simulink model "RmsConverterController_R2014b"  (R2014b)
settings: Solver=ode2  SolverMode=SingleTasking  StartTime=0.0  StopTime=10.0  FixedStep=2e-5  RelTol=1e-3
libraries: simulink x4, powerlib_meascontrol x2
settings Model: CovMetricSettings=dwe  CovHtmlReporting=off  covSaveCumulativeToWorkspaceVar=off  CovSaveSingleToWorkspaceVar=off  CovExternalEMLEnable=on  CovSFcnEnable=on  Creator=sandroni  LastModifiedBy=carlo
settings DataIOCC: LimitDataPoints=off  SaveFormat=StructureWithTime
settings DebuggingCC: SolverPrmCheckMsg=none  FrameProcessingCompatibilityMsg=error  SFUnexpectedBacktrackingDiag=error  SFNoUnconditionalDefaultTransitionDiag=error
settings HardwareCC: ProdBitPerPointer=64  ProdLargestAtomicFloat=Float  ProdIntDivRoundTo=Zero  ProdEndianess=LittleEndian  ProdHWDeviceType=Specified  TargetLongLongMode=on  TargetIntDivRoundTo=Zero  TargetEndianess=LittleEndian  TargetHWDeviceType=MATLAB Host  ProdEqTarget=off
settings ModelReferenceCC: PropagateSignalLabelsOutOfModel=on
settings RTWCC: SystemTargetFile=rtwsfcnfmi.tlc  TemplateMakefile=rtwsfcnfmi_tmf  Description=S-Function Target with Functional Mockup Interface (FMI)  ProcessScript=rtwsfcnfmi_make_rtw_hook
settings STFCustomTargetCC: ModelReferenceCompliant=off  CompOptLevelCompliant=on  GeneratePreprocessorConditionals=Disable all  MATLABClassNameForMDSCustomization=Simulink.SoftwareTarget.TargetSpecificTriggerConfigurationBase  SystemTargetFile=rtwsfcnfmi.tlc

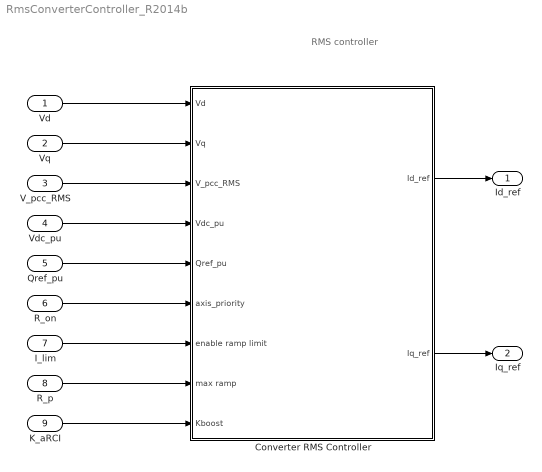
== system RmsConverterController_R2014b ==
  note: RMS controller
  Vd : Inport
  Vq : Inport  Port=2
  V_pcc_RMS : Inport  Port=3
  Vdc_pu : Inport  Port=4
  Qref_pu : Inport  Port=5
  R_on : Inport  Port=6
  I_lim : Inport  Port=7
  R_p : Inport  Port=8
  K_aRCI : Inport  Port=9
  Converter RMS Controller : Subsystem  mask(Converter RMS Controller){Kp_dc=1.1, Ki_dc=27.5, Kp_Var=1, Ki_Var=100, P0_pu=0.85, Fnom=50, Ts=2e-5}
      mask prompts: Kp_dc "DC voltage regulator proportional parameter [Kp]"; Ki_dc "DC voltage regulator integral parameter [Ki]"; Kp_Var "PCC voltage regulator proportional parameter [Kp]"; Ki_Var "PCC voltage regulator integral parameter [Ki]"; P0_pu "Initial Active Power [pu]"; Fnom "Nominal frequency [Hz]"; Ts "Sample Time [s]"
      mask init:
      | Imax_grid_conv = 1.1;
  Id_ref : Outport
  Iq_ref : Outport  Port=2
  wires:
  Qref_pu/1 -> Converter RMS Controller/5(Qref_pu)
  V_pcc_RMS/1 -> Converter RMS Controller/3(V_pcc_RMS)
  K_aRCI/1 -> Converter RMS Controller/9(Kboost)
  R_on/1 -> Converter RMS Controller/6(axis_priority)
  R_p/1 -> Converter RMS Controller/8(max ramp)
  I_lim/1 -> Converter RMS Controller/7(enable ramp limit)
  Converter RMS Controller/1(Id_ref) -> Id_ref/1
  Converter RMS Controller/2(Iq_ref) -> Iq_ref/1
  Vq/1 -> Converter RMS Controller/2(Vq)
  Vdc_pu/1 -> Converter RMS Controller/4(Vdc_pu)
  Vd/1 -> Converter RMS Controller/1(Vd)

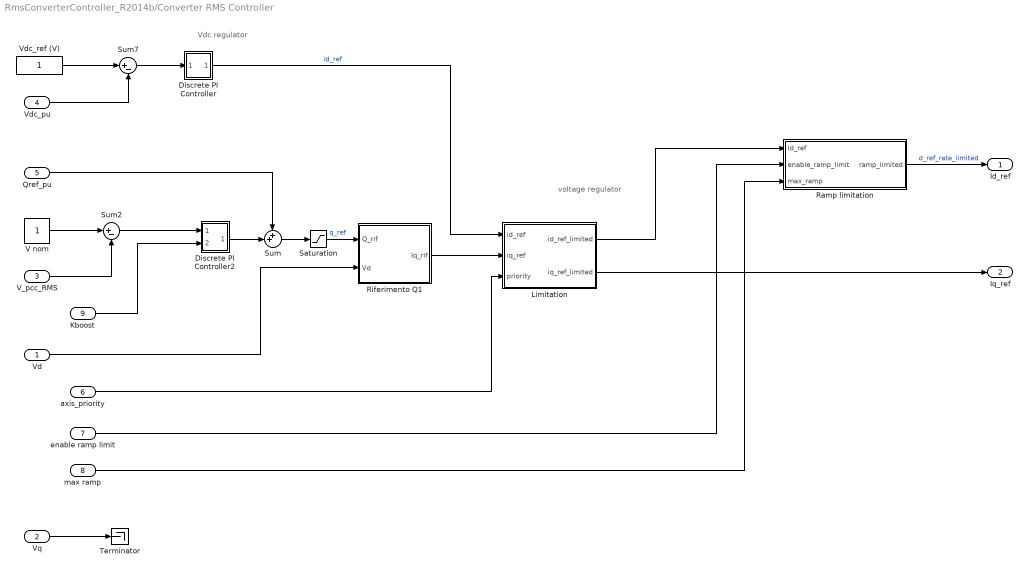
== system RmsConverterController_R2014b/Converter RMS Controller ==
  note: Vdc regulator
  note: voltage regulator
  Vd : Inport
  Vq : Inport  Port=2
  V_pcc_RMS : Inport  Port=3
  Vdc_pu : Inport  Port=4
  Qref_pu : Inport  Port=5
  axis_priority : Inport  Port=6
  enable ramp limit : Inport  Port=7
  max ramp : Inport  Port=8
  Kboost : Inport  Port=9
  Discrete PI Controller : Subsystem  DialogController=POWERSYS.PowerSysDialog  mask(Discrete PI Controller){Kp=Kp_dc, Ki=Ki_dc, Par_Limits=[1 -1]*Imax_grid_conv, Init=-P0_pu, Ts=Ts}
      mask prompts: Kp "Proportional gain (Kp):"; Ki "Integral gain (Ki):"; Par_Limits "Output limits: [ Upper   Lower ]"; Init "Output initial value:"; Ts "Sample time:"
      mask help: This block implements a discrete PI controller.
      mask init:
      | UpperLimit=Par_Limits(1);
      | LowerLimit=Par_Limits(2);
      | power_initmask();
      mask Help: This block is part of a subset of blocks in the Extras library that does not have documentation associated with it, other than the block mask description.
      mask Display: disp('PI');
  Discrete PI Controller2 : Subsystem  DialogController=POWERSYS.PowerSysDialog  mask(Discrete PI Controller){Kp=Kp_Var, Ki=Ki_Var, Par_Limits=[1 -1], Init=0, Ts=Ts}
      mask prompts: Kp "Proportional gain (Kp):"; Ki "Integral gain (Ki):"; Par_Limits "Output limits: [ Upper   Lower ]"; Init "Output initial value:"; Ts "Sample time:"
      mask help: This block implements a discrete PI controller.
      mask init:
      | UpperLimit=Par_Limits(1);
      | LowerLimit=Par_Limits(2);
      | power_initmask();
      mask Help: This block is part of a subset of blocks in the Extras library that does not have documentation associated with it, other than the block mask description.
      mask Display: disp('PI');
  Limitation : Subsystem
  Ramp limitation : Subsystem
  Riferimento Q1 : Subsystem
  Saturation : Saturate  UpperLimit=1  LowerLimit=-1
  Sum : Sum  Inputs=++|
  Sum2 : Sum  Inputs=|+-  SaturateOnIntegerOverflow=on  InputSameDT=on  OutDataTypeStr=Inherit: Same as first input
  Sum7 : Sum  Inputs=|+-  SaturateOnIntegerOverflow=on  InputSameDT=on  OutDataTypeStr=Inherit: Same as first input
  Terminator : Terminator
  V nom : Constant
  Vdc_ref (V) : Constant
  Id_ref : Outport
  Iq_ref : Outport  Port=2
  wires:
  Sum7/1 -> Discrete PI Controller/1(Error)
  Vdc_ref (V)/1 -> Sum7/1
  Vd/1 -> Riferimento Q1/2(Vd)
  Sum2/1 -> Discrete PI Controller2/1(Error)
  V nom/1 -> Sum2/1
  V_pcc_RMS/1 -> Sum2/2
  Qref_pu/1 -> Sum/1
  Sum/1 -> Saturation/1
  Discrete PI Controller2/1(Out) -> Sum/2
  Saturation/1 -> Riferimento Q1/1(Q_rif)  "q_ref"
  Vdc_pu/1 -> Sum7/2
  Kboost/1 -> Discrete PI Controller2/2(K_aRCI)
  axis_priority/1 -> Limitation/3(priority)
  Riferimento Q1/1(Iq_rif) -> Limitation/2(iq_ref)
  Discrete PI Controller/1(Out) -> Limitation/1(id_ref)  "id_ref"
  Limitation/2(iq_ref_limited) -> Iq_ref/1
  Ramp limitation/1(ramp_limited) -> Id_ref/1  "d_ref_rate_limited"
  Limitation/1(id_ref_limited) -> Ramp limitation/1(Id_ref)
  enable ramp limit/1 -> Ramp limitation/2(enable_ramp_limit)
  max ramp/1 -> Ramp limitation/3(max_ramp)
  Vq/1 -> Terminator/1

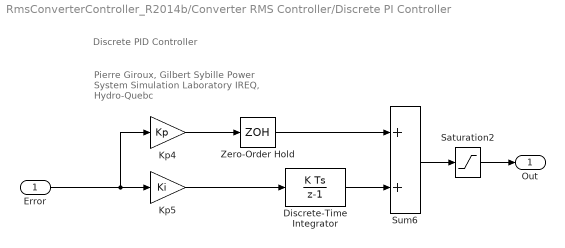
== system RmsConverterController_R2014b/Converter RMS Controller/Discrete PI Controller ==
  note: Discrete PID Controller
  note: Pierre Giroux, Gilbert Sybille
      | Power System Simulation Laboratory
      | IREQ, Hydro-Quebc
  Error : Inport  SampleTime=Ts
  Discrete-Time Integrator : DiscreteIntegrator  InitialCondition=Init  SampleTime=Ts  LimitOutput=on  UpperSaturationLimit=UpperLimit  LowerSaturationLimit=LowerLimit
  Kp4 : Gain  Gain=Kp  SampleTime=Ts  SaturateOnIntegerOverflow=on  OutDataTypeStr=Inherit: Same as input  ParamDataTypeStr=Inherit: Same as input
  Kp5 : Gain  Gain=Ki  SampleTime=Ts  SaturateOnIntegerOverflow=on  OutDataTypeStr=Inherit: Same as input  ParamDataTypeStr=Inherit: Same as input
  Saturation2 : Saturate  UpperLimit=UpperLimit  LowerLimit=LowerLimit  SampleTime=Ts
  Sum6 : Sum  SampleTime=Ts  SaturateOnIntegerOverflow=on  InputSameDT=on  OutDataTypeStr=Inherit: Same as first input
  Zero-Order Hold : ZeroOrderHold  SampleTime=Ts
  Out : Outport  SampleTime=Ts  InitialOutput=0
  wires:
  Zero-Order Hold/1 -> Sum6/1
  Saturation2/1 -> Out/1
  Discrete-Time Integrator/1 -> Sum6/2
  Kp4/1 -> Zero-Order Hold/1
  Kp5/1 -> Discrete-Time Integrator/1
  Sum6/1 -> Saturation2/1
  Error/1 -> Kp5/1, Kp4/1

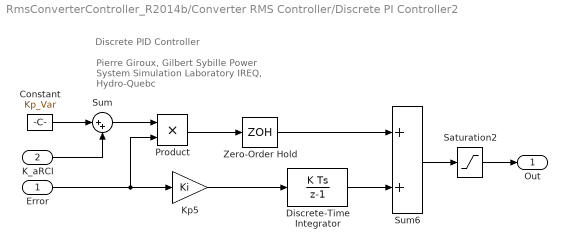
== system RmsConverterController_R2014b/Converter RMS Controller/Discrete PI Controller2 ==
  note: Discrete PID Controller
  note: Pierre Giroux, Gilbert Sybille
      | Power System Simulation Laboratory
      | IREQ, Hydro-Quebc
  Error : Inport  SampleTime=Ts
  K_aRCI : Inport  Port=2  SampleTime=Ts
  Constant : Constant  Value=Kp_Var
  Discrete-Time Integrator : DiscreteIntegrator  InitialCondition=Init  SampleTime=Ts  LimitOutput=on  UpperSaturationLimit=UpperLimit  LowerSaturationLimit=LowerLimit
  Kp5 : Gain  Gain=Ki  SampleTime=Ts  SaturateOnIntegerOverflow=on  OutDataTypeStr=Inherit: Same as input  ParamDataTypeStr=Inherit: Same as input
  Product : Product
  Saturation2 : Saturate  UpperLimit=UpperLimit  LowerLimit=LowerLimit  SampleTime=Ts
  Sum : Sum  Inputs=|++
  Sum6 : Sum  SampleTime=Ts  SaturateOnIntegerOverflow=on  InputSameDT=on  OutDataTypeStr=Inherit: Same as first input
  Zero-Order Hold : ZeroOrderHold  SampleTime=Ts
  Out : Outport  SampleTime=Ts  InitialOutput=0
  wires:
  Zero-Order Hold/1 -> Sum6/1
  Saturation2/1 -> Out/1
  Discrete-Time Integrator/1 -> Sum6/2
  Sum6/1 -> Saturation2/1
  Error/1 -> Kp5/1, Product/2
  K_aRCI/1 -> Sum/2
  Product/1 -> Zero-Order Hold/1
  Sum/1 -> Product/1
  Constant/1 -> Sum/1
  Kp5/1 -> Discrete-Time Integrator/1

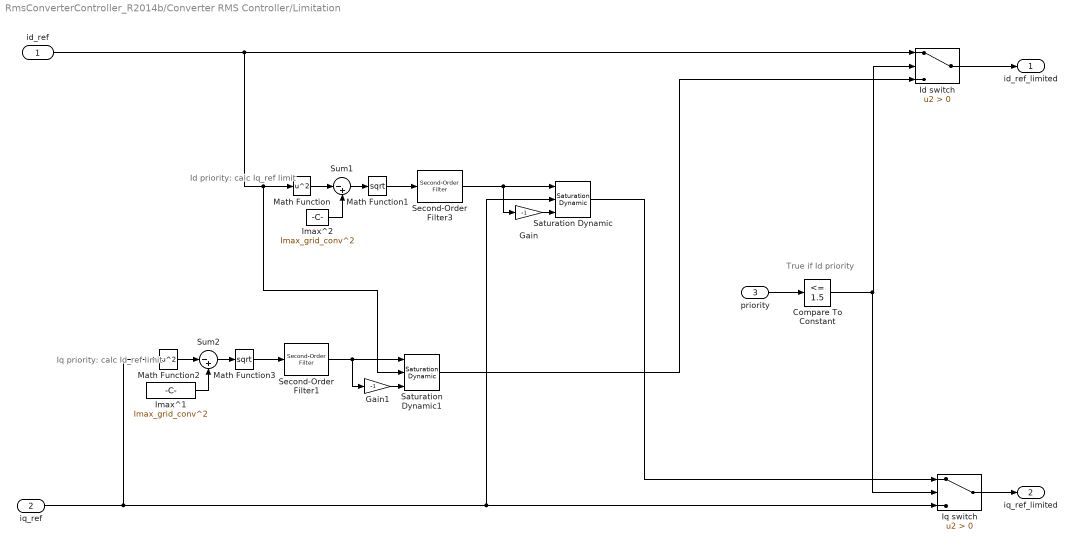
== system RmsConverterController_R2014b/Converter RMS Controller/Limitation ==
  note: Id priority:
      | calc Iq_ref limit
  note: True if Id priority
  note: Iq priority:
      | calc Id_ref limit
  id_ref : Inport
  iq_ref : Inport  Port=2
  priority : Inport  Port=3
  Compare To Constant : simulink/Logic and Bit Operations/Compare To Constant  relop=<=  const=1.5  OutDataTypeStr=boolean
  Gain : Gain  Gain=-1
  Gain1 : Gain  Gain=-1
  Id switch : Switch  Criteria=u2 > Threshold
  Imax^1 : Constant  Value=Imax_grid_conv^2
  Imax^2 : Constant  Value=Imax_grid_conv^2
  Iq switch : Switch  Criteria=u2 > Threshold
  Math Function : Math  Operator=square  SaturateOnIntegerOverflow=on
  Math Function1 : Math  Operator=sqrt  SaturateOnIntegerOverflow=on
  Math Function2 : Math  Operator=square  SaturateOnIntegerOverflow=on
  Math Function3 : Math  Operator=sqrt  SaturateOnIntegerOverflow=on
  Saturation Dynamic : simulink/Discontinuities/Saturation Dynamic  OutMin=[]  OutMax=[]  OutDataTypeStr=Inherit: Same as second input  OutDataType=fixdt(1, 16)  OutScaling=2^-10  DoSatur=off
  Saturation Dynamic1 : simulink/Discontinuities/Saturation Dynamic  OutMin=[]  OutMax=[]  OutDataTypeStr=Inherit: Same as second input  OutDataType=fixdt(1, 16)  OutScaling=2^-10  DoSatur=off
  Second-Order Filter1 : powerlib_meascontrol/Filters/Second-Order Filter  FilterType=Lowpass  Fo=Fnom  Zeta=1  Ts=Ts  Initialize=on  Vac_Init="[0,  0,  50]"  Vdc_Init=Imax_grid_conv  PlotResponse=off  FreqRange=[0, 500, 1]
  Second-Order Filter3 : powerlib_meascontrol/Filters/Second-Order Filter  FilterType=Lowpass  Fo=Fnom  Zeta=1  Ts=Ts  Initialize=on  Vac_Init="[0,  0,  50]"  Vdc_Init=sqrt(Imax_grid_conv^2-P0_pu^2)  PlotResponse=off  FreqRange=[0, 500, 1]
  Sum1 : Sum  Inputs=|-+  SaturateOnIntegerOverflow=on  InputSameDT=on  OutDataTypeStr=Inherit: Same as first input
  Sum2 : Sum  Inputs=|-+  SaturateOnIntegerOverflow=on  InputSameDT=on  OutDataTypeStr=Inherit: Same as first input
  id_ref_limited : Outport
  iq_ref_limited : Outport  Port=2
  wires:
  Imax^2/1 -> Sum1/2
  Math Function/1 -> Sum1/1
  Sum1/1 -> Math Function1/1
  Gain/1 -> Saturation Dynamic/3
  Math Function1/1 -> Second-Order Filter3/1
  priority/1 -> Compare To Constant/1
  Compare To Constant/1 -> Iq switch/2, Id switch/2
  Saturation Dynamic/1 -> Iq switch/1
  Imax^1/1 -> Sum2/2
  Math Function2/1 -> Sum2/1
  Sum2/1 -> Math Function3/1
  Gain1/1 -> Saturation Dynamic1/3
  Math Function3/1 -> Second-Order Filter1/1
  Saturation Dynamic1/1 -> Id switch/3
  Id switch/1 -> id_ref_limited/1
  Iq switch/1 -> iq_ref_limited/1
  id_ref/1 -> Saturation Dynamic1/2, Math Function/1, Id switch/1
  iq_ref/1 -> Math Function2/1, Saturation Dynamic/2, Iq switch/3
  Second-Order Filter3/1 -> Gain/1, Saturation Dynamic/1
  Second-Order Filter1/1 -> Gain1/1, Saturation Dynamic1/1

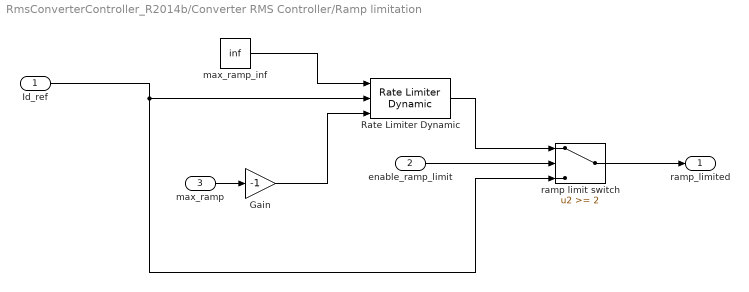
== system RmsConverterController_R2014b/Converter RMS Controller/Ramp limitation ==
  Id_ref : Inport
  enable_ramp_limit : Inport  Port=2
  max_ramp : Inport  Port=3
  Gain : Gain  Gain=-1
  Rate Limiter Dynamic : simulink/Discontinuities/Rate Limiter Dynamic
  max_ramp_inf : Constant  Value=inf
  ramp limit switch : Switch  Threshold=2
  ramp_limited : Outport
  wires:
  ramp limit switch/1 -> ramp_limited/1
  Id_ref/1 -> ramp limit switch/3, Rate Limiter Dynamic/2
  enable_ramp_limit/1 -> ramp limit switch/2
  Rate Limiter Dynamic/1 -> ramp limit switch/1
  max_ramp_inf/1 -> Rate Limiter Dynamic/1
  max_ramp/1 -> Gain/1
  Gain/1 -> Rate Limiter Dynamic/3

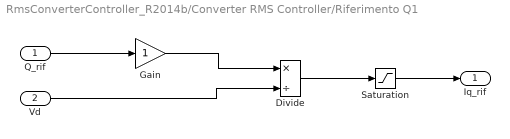
== system RmsConverterController_R2014b/Converter RMS Controller/Riferimento Q1 ==
  Q_rif : Inport
  Vd : Inport  Port=2
  Divide : Product  Inputs=*/
  Gain : Gain
  Saturation : Saturate  UpperLimit=1  LowerLimit=-1
  Iq_rif : Outport
  wires:
  Vd/1 -> Divide/2
  Gain/1 -> Divide/1
  Q_rif/1 -> Gain/1
  Divide/1 -> Saturation/1
  Saturation/1 -> Iq_rif/1
